simulink model "bouncing_ball"  (R2022b)
settings: Solver=ode1  StartTime=0.0  StopTime=20  FixedStep=0.001  RelTol=1e-3
libraries: simulink x1
settings Model: Creator=user  LastModifiedBy=user

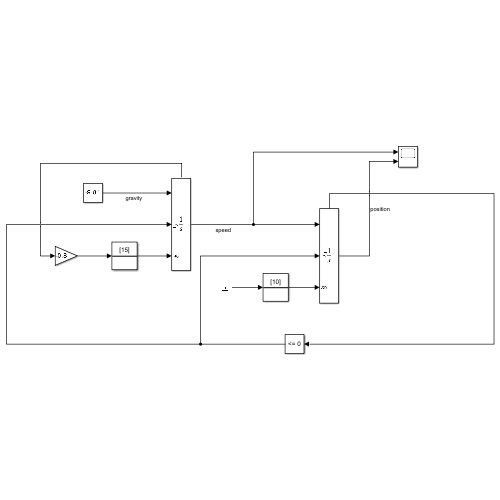
[thumbnail: Simulink's stored preview of the top-level diagram]
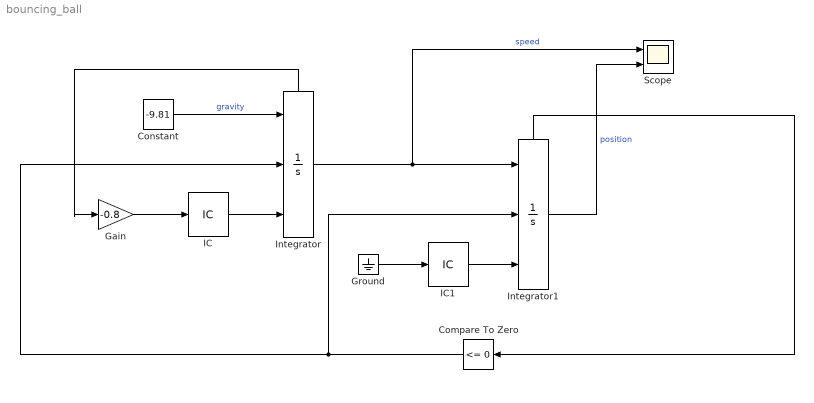
== system bouncing_ball ==
  Compare To Zero : simulink/Logic and Bit Operations/Compare To Zero  relop=<=  OutDataTypeStr=boolean
  Constant : Constant  Value=-9.81
  Gain : Gain  Gain=-0.8
  Ground : Ground
  IC : InitialCondition  Value=15
  IC1 : InitialCondition  Value=10
  Integrator : Integrator  ExternalReset=rising  InitialConditionSource=external  InitialCondition=15  ShowStatePort=on
  Integrator1 : Integrator  ExternalReset=rising  InitialConditionSource=external  InitialCondition=10  ShowStatePort=on
  Scope : Scope  NumInputPorts=2
  wires:
  Constant/1 -> Integrator/1  "gravity"
  Integrator/1 -> Scope/1, Integrator1/1  "speed"
  Integrator1/1 -> Scope/2  "position"
  Integrator1/State -> Compare To Zero/1
  Compare To Zero/1 -> Integrator/2, Integrator1/2
  IC/1 -> Integrator/3
  IC1/1 -> Integrator1/3
  Ground/1 -> IC1/1
  Integrator/State -> Gain/1
  Gain/1 -> IC/1
